simulink library "Surface_Profile_Axle2_zx"  (R2025a)
settings: Solver=VariableStepAuto  StartTime=0.0  StopTime=10.0  RelTol=1e-3
Description:
  | Simscape Vehicle Templates Library
  | 
  | Copyright 2018-2025 The MathWorks, Inc.
settings Model: Creator=smiller  LastModifiedBy=smiller
settings ModelReferenceCC: EnableRefExpFcnMdlSchedulingChecks=on
settings RTWCC: GPUComputeCapability=3.5

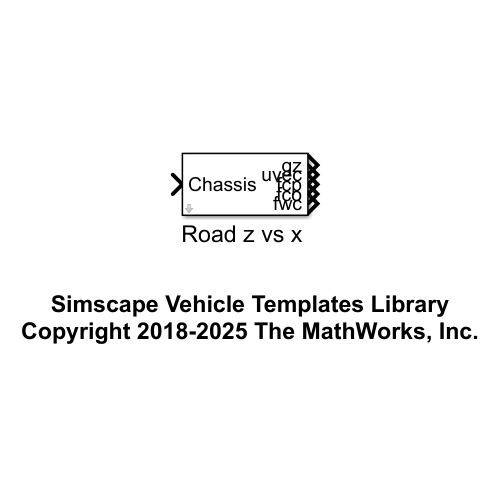
[thumbnail: Simulink's stored preview of the top-level diagram]
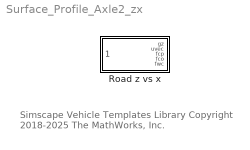
== system Surface_Profile_Axle2_zx ==
  note: Simscape Vehicle Templates Library
      | Copyright 2018-2025 The MathWorks, Inc.
  "Road z vs x " : Subsystem  VariantControl=Plateau  mask{dist_x=flipud(Scene.RDF_Plateau.Road.extr_data_L(109:end,1)), height_z=flipud(Scene.RDF_Plateau.Road.extr_data_L(109:end,2))}
      mask prompts: dist_x "Distance vector [x] (m)"; height_z "Height vector [z] (m)"
      mask init:
      | pitch_rd = atan2(circshift(height_z,-2)-circshift(height_z,2),circshift(dist_x,-2)-circshift(dist_x,2));
      | pitch_rd(1:2) = pitch_rd(3);
      | pitch_rd(end-1:end) = pitch_rd(end-2);

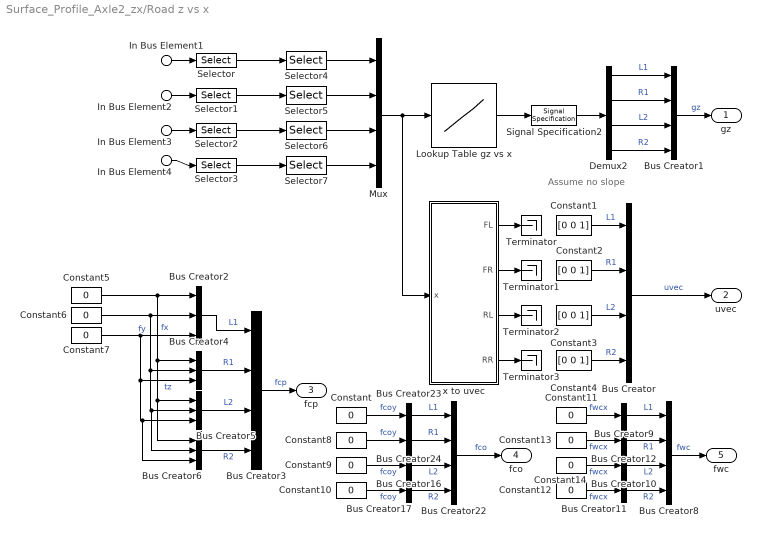
== system Surface_Profile_Axle2_zx/Road z vs x  ==
  note: Assume no slope
  In Bus Element1 : Inport  PortName=Chassis  Element=WhlL1.xyz
  In Bus Element2 : Inport  PortName=Chassis  Element=WhlR1.xyz
  In Bus Element3 : Inport  PortName=Chassis  Element=WhlL2.xyz
  In Bus Element4 : Inport  PortName=Chassis  Element=WhlR2.xyz
  Bus Creator{,1,3,8,22} (5 alike) : BusCreator  Inputs=4
  Bus Creator{9..12,16..17,23..24} (8 alike) : BusCreator  Inputs=1
  Bus Creator{2,4..6} (4 alike) : BusCreator  Inputs=3
  Constant{,5..14} (11 alike) : Constant  Value=0
  Constant{1..4} (4 alike) : Constant  Value=[0 0 1]
  Demux2 : Demux
  Lookup Table gz vs x : Lookup_n-D  NumberOfTableDimensions=1  BreakpointsForDimension1=dist_x  Table=height_z  InternalRulePriority=Speed  RndMeth=Simplest
  Mux : Mux
  Selector{,1..3} (4 alike) : Selector  InputPortWidth=3  IndexOptions=Index vector (dialog)  Indices=[1 2]  OutputSizes=1
  Selector{4..7} (4 alike) : Selector  InputPortWidth=2  IndexOptions=Index vector (dialog)  Indices=1  OutputSizes=1
  Signal Specification2 : SignalSpecification  Unit=m
  Terminator{,1..3} (4 alike) : Terminator
  x to uvec : Subsystem
  gz : Outport  VectorParamsAs1DForOutWhenUnconnected=off
  uvec : Outport  Port=2  VectorParamsAs1DForOutWhenUnconnected=off
  fcp : Outport  Port=3  VectorParamsAs1DForOutWhenUnconnected=off
  fco : Outport  Port=4  VectorParamsAs1DForOutWhenUnconnected=off
  fwc : Outport  Port=5  VectorParamsAs1DForOutWhenUnconnected=off
  wires:
  Constant7/1 -> Bus Creator2/3, Bus Creator4/3, Bus Creator5/3, Bus Creator6/3  "tz"
  Constant6/1 -> Bus Creator2/2, Bus Creator4/2, Bus Creator5/2, Bus Creator6/2  "fy"
  Constant5/1 -> Bus Creator2/1, Bus Creator4/1, Bus Creator5/1, Bus Creator6/1  "fx"
  Bus Creator6/1 -> Bus Creator3/4  "R2"
  Bus Creator5/1 -> Bus Creator3/3  "L2"
  Bus Creator2/1 -> Bus Creator3/1  "L1"
  Bus Creator4/1 -> Bus Creator3/2  "R1"
  Bus Creator3/1 -> fcp/1  "fcp"
  Constant4/1 -> Bus Creator/4  "R2"
  Constant3/1 -> Bus Creator/3  "L2"
  Constant2/1 -> Bus Creator/2  "R1"
  x to uvec/4(RR) -> Terminator3/1
  x to uvec/3(RL) -> Terminator2/1
  x to uvec/2(FR) -> Terminator1/1
  x to uvec/1(FL) -> Terminator/1
  Constant1/1 -> Bus Creator/1  "L1"
  Bus Creator/1 -> uvec/1  "uvec"
  Bus Creator1/1 -> gz/1  "gz"
  Demux2/4 -> Bus Creator1/4  "R2"
  Demux2/1 -> Bus Creator1/1  "L1"
  Demux2/2 -> Bus Creator1/2  "R1"
  Signal Specification2/1 -> Demux2/1
  Demux2/3 -> Bus Creator1/3  "L2"
  In Bus Element3/1 -> Selector2/1
  In Bus Element1/1 -> Selector/1
  In Bus Element2/1 -> Selector1/1
  In Bus Element4/1 -> Selector3/1
  Selector/1 -> Selector4/1
  Selector1/1 -> Selector5/1
  Selector2/1 -> Selector6/1
  Selector3/1 -> Selector7/1
  Selector7/1 -> Mux/4
  Selector6/1 -> Mux/3
  Selector5/1 -> Mux/2
  Selector4/1 -> Mux/1
  Mux/1 -> Lookup Table gz vs x/1, x to uvec/1(x)
  Lookup Table gz vs x/1 -> Signal Specification2/1
  Bus Creator12/1 -> Bus Creator8/2  "R1"
  Bus Creator24/1 -> Bus Creator22/2  "R1"
  Bus Creator10/1 -> Bus Creator8/3  "L2"
  Bus Creator9/1 -> Bus Creator8/1  "L1"
  Bus Creator16/1 -> Bus Creator22/3  "L2"
  Bus Creator22/1 -> fco/1  "fco"
  Bus Creator23/1 -> Bus Creator22/1  "L1"
  Bus Creator17/1 -> Bus Creator22/4  "R2"
  Constant8/1 -> Bus Creator24/1  "fcoy"
  Constant10/1 -> Bus Creator17/1  "fcoy"
  Constant9/1 -> Bus Creator16/1  "fcoy"
  Constant12/1 -> Bus Creator11/1  "fwcx"
  Constant14/1 -> Bus Creator10/1  "fwcx"
  Constant13/1 -> Bus Creator12/1  "fwcx"
  Bus Creator8/1 -> fwc/1  "fwc"
  Constant11/1 -> Bus Creator9/1  "fwcx"
  Constant/1 -> Bus Creator23/1  "fcoy"
  Bus Creator11/1 -> Bus Creator8/4  "R2"

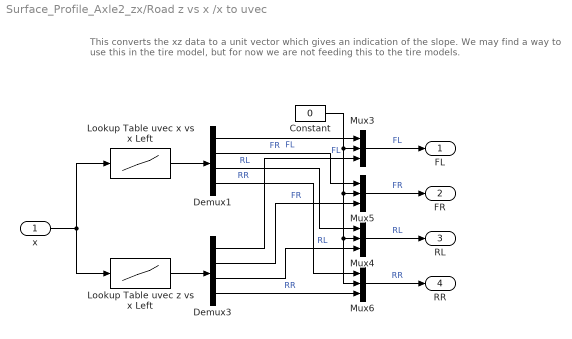
== system Surface_Profile_Axle2_zx/Road z vs x /x to uvec ==
  note: This converts the xz data to a unit vector which gives an indication of the slope. We may find a way to use this in the tire model, but for now we are not feeding this to the tire models.
  x : Inport
  Constant : Constant  Value=0
  Demux1 : Demux
  Demux3 : Demux
  Lookup Table uvec x vs x Left : Lookup_n-D  NumberOfTableDimensions=1  BreakpointsForDimension1=dist_x  Table=sin(pitch_rd)  InternalRulePriority=Speed  RndMeth=Simplest
  Lookup Table uvec z vs x Left : Lookup_n-D  NumberOfTableDimensions=1  BreakpointsForDimension1=dist_x  Table=cos(pitch_rd)  InternalRulePriority=Speed  RndMeth=Simplest
  Mux{3..6} (4 alike) : Mux  Inputs=3
  FL : Outport  VectorParamsAs1DForOutWhenUnconnected=off
  FR : Outport  Port=2  VectorParamsAs1DForOutWhenUnconnected=off
  RL : Outport  Port=3  VectorParamsAs1DForOutWhenUnconnected=off
  RR : Outport  Port=4  VectorParamsAs1DForOutWhenUnconnected=off
  wires:
  Mux4/1 -> RL/1  "RL"
  Demux3/1 -> Mux3/3  "FL"
  Demux1/4 -> Mux6/1  "RR"
  Demux3/4 -> Mux6/3  "RR"
  Demux3/2 -> Mux5/3  "FR"
  Demux1/1 -> Mux3/1  "FL"
  Mux5/1 -> FR/1  "FR"
  Demux3/3 -> Mux4/3  "RL"
  Lookup Table uvec x vs x Left/1 -> Demux1/1
  Constant/1 -> Mux3/2, Mux5/2, Mux4/2, Mux6/2
  Mux3/1 -> FL/1  "FL"
  Lookup Table uvec z vs x Left/1 -> Demux3/1
  Demux1/3 -> Mux4/1  "RL"
  Demux1/2 -> Mux5/1  "FR"
  Mux6/1 -> RR/1  "RR"
  x/1 -> Lookup Table uvec z vs x Left/1, Lookup Table uvec x vs x Left/1
